simulink model "Filter_Subsytem"  (R2020b)
settings: Solver=VariableStepAuto  StartTime=0.0  StopTime=10.0  RelTol=1e-3
settings Model: Creator=Shantam Garg  LastModifiedBy=Shantam Garg
settings DataIOCC: SaveOutput=off  SaveTime=off

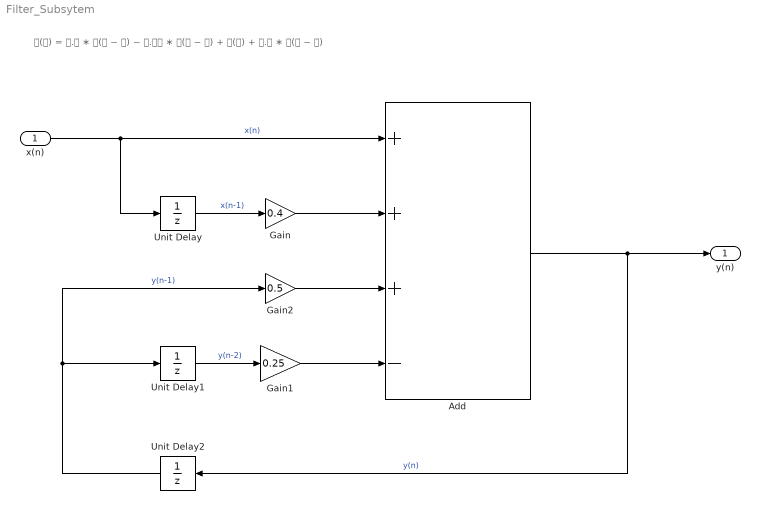
== system Filter_Subsytem ==
  note: 𝐲(𝐧) = 𝟎.𝟓 ∗ 𝐲(𝐧 − 𝟏) − 𝟎.𝟐𝟓 ∗ 𝐲(𝐧 − 𝟐) + 𝐱(𝐧) + 𝟎.𝟒 ∗ 𝐱(𝐧 − 𝟏)
  x(n) : Inport  OutDataTypeStr=double  PortDimensions=1  SampleTime=[0,1]
  Add : Sum  Inputs=+++-
  Gain : Gain  Gain=0.4
  Gain1 : Gain  Gain=0.25
  Gain2 : Gain  Gain=0.5
  Unit Delay : UnitDelay  SampleTime=-1  HasFrameUpgradeWarning=on
  Unit Delay1 : UnitDelay  SampleTime=-1  HasFrameUpgradeWarning=on
  Unit Delay2 : UnitDelay  SampleTime=-1  HasFrameUpgradeWarning=on
  y(n) : Outport  OutDataTypeStr=double  PortDimensions=1  SampleTime=[0,1]
  wires:
  Gain2/1 -> Add/3
  Add/1 -> Unit Delay2/1, y(n)/1  "y(n)"
  Unit Delay1/1 -> Gain1/1  "y(n-2)"
  x(n)/1 -> Unit Delay/1, Add/1  "x(n)"
  Unit Delay/1 -> Gain/1  "x(n-1)"
  Unit Delay2/1 -> Unit Delay1/1, Gain2/1  "y(n-1)"
  Gain/1 -> Add/2
  Gain1/1 -> Add/4
